simulink model "AnalogeSignalProcessing"  (R2023b)
settings: Solver=VariableStepAuto  StartTime=0.0  StopTime=10.0  RelTol=1e-3
PostLoadFcn:
  | if any(exist('dsrtsu_mdlpostloadfcn', 'file') ~= 0), dsrtsu_mdlpostloadfcn('Execute', bdroot); end
InitFcn:
  | , if any(exist('dsmpb_private', 'file') ~= 0), dsmpb_private('dsmpb_mdlclblib', 'Init', bdroot); end,
libraries: dsmpblib x2
PreSaveFcn:
  | , if any(exist('dsmpb_private', 'file') ~= 0), dsmpb_private('dsmpb_mdlclblib', 'PreSave', bdroot); end,
CloseFcn:
  | , if any(exist('dsmpb_private', 'file') ~= 0), dsmpb_private('dsmpb_mdlclblib', 'Close', bdroot); end,
settings Model: DSMPB_ID_DATA={'13',struct('BlockId','c6f1ea6c-9ae7-4009-922d-066e0d717a3f','SignalIds',{{'b7d7c5cf-bc63-43a8-8148-9b649da1d95a'}}),'14',struct('BlockId','f4325053-4ade-4a68-95b5-ca9ce18cf876','SignalIds',{{'690a07a9-1a1a-403e-8bb8-196457143d42'}})}  Creator=MURTI  LastModifiedBy=MURTI

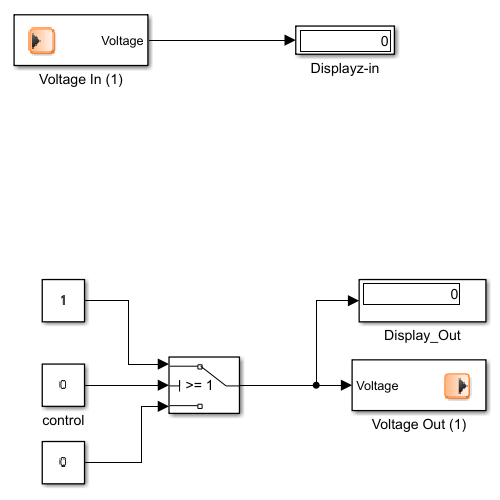
[thumbnail: Simulink's stored preview of the top-level diagram]
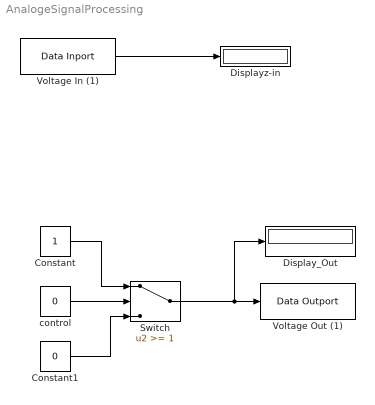
== system AnalogeSignalProcessing ==
  Constant : Constant
  Constant1 : Constant  Value=0
  Display_Out : Display
  Displayz-in : Display
  Switch : Switch  Threshold=1  SaturateOnIntegerOverflow=off  InputSameDT=off
  Voltage In (1) : dsmpblib/Data Inport  Priority=10000
      settings: SourceProductName=dSPACE Model Interface Package for Simulink (MIPS)
  Voltage Out (1) : dsmpblib/Data Outport  Priority=-10000
      settings: SourceProductName=dSPACE Model Interface Package for Simulink (MIPS)
  control : Constant  Value=0
  wires:
  control/1 -> Switch/2
  Voltage In (1)/1 -> Displayz-in/1
  Constant1/1 -> Switch/3
  Constant/1 -> Switch/1
  Switch/1 -> Voltage Out (1)/1, Display_Out/1
